simulink model "noise"  (R2016a)
settings: Solver=VariableStepAuto  StartTime=0.0  StopTime=10.0  RelTol=1e-3
libraries: dspsrcs4 x1
settings Model: Creator=Atulya  LastModifiedBy=Atulya

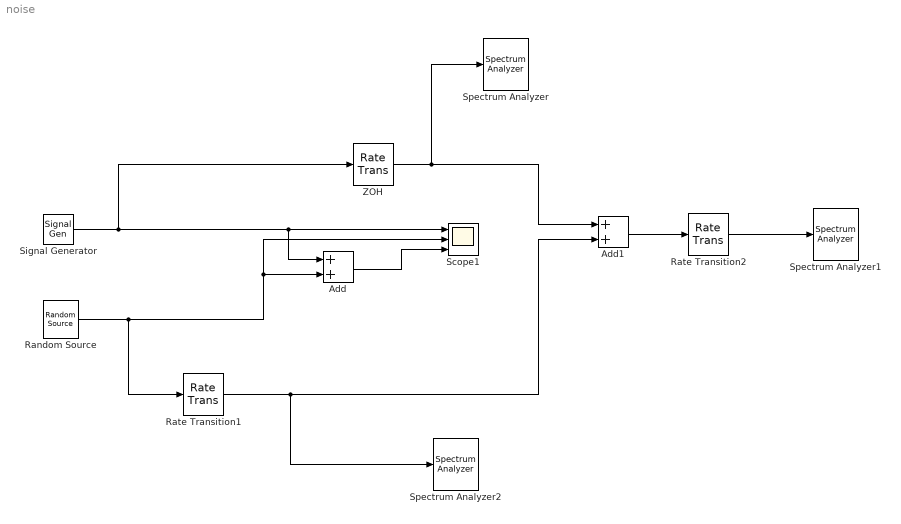
== system noise ==
  Add : Sum
  Add1 : Sum
  Random Source : dspsrcs4/Random Source  SrcType=Gaussian  NormMethod=Ziggurat  CltLength=12  MinVal=0  MaxVal=1  MeanVal=0.1  VarVal=0.02  RepMode=Repeatable  rawSeed=1  IsInherit=off  SampMode=Continuous  SampTime=1  SampFrame=1  DataType=Double  OutComplex=Real  OutputFrames=off
  Rate Transition1 : RateTransition  X0=0.001
  Rate Transition2 : RateTransition  OutPortSampleTime=0.001
  Scope1 : Scope  NumInputPorts=3
  Signal Generator : SignalGenerator  Amplitude=0.1  Frequency=10
  Spectrum Analyzer : SpectrumAnalyzer
  Spectrum Analyzer1 : SpectrumAnalyzer
  Spectrum Analyzer2 : SpectrumAnalyzer
  ZOH : RateTransition  OutPortSampleTime=0.001
  wires:
  Signal Generator/1 -> ZOH/1, Add/1, Scope1/1
  Random Source/1 -> Rate Transition1/1, Add/2, Scope1/2
  Add/1 -> Scope1/3
  ZOH/1 -> Spectrum Analyzer/1, Add1/1
  Rate Transition1/1 -> Spectrum Analyzer2/1, Add1/2
  Add1/1 -> Rate Transition2/1
  Rate Transition2/1 -> Spectrum Analyzer1/1
